simulink model "NAO68"  (R2021b)
settings: Solver=VariableStepAuto  StartTime=0.0  StopTime=2
undefined symbols (not defined in the file): foot_z, X, Y, Z
libraries: sm_lib x258, nesl_utility x25, Contact_Forces_Lib x3, simulink x1
(part 6 of 6)

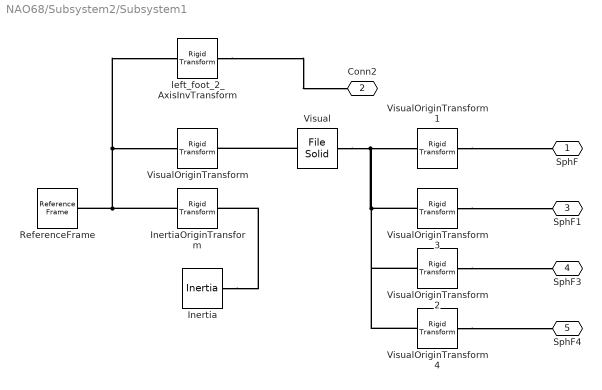
== system NAO68/Subsystem2/Subsystem1 ==
  Inertia : sm_lib/Body Elements/Inertia  InertiaType=Custom  Mass=2.1641e-17  MassUnits=kg  CenterOfMass=[0, 0, 0]  CenterOfMassUnits=m  MomentsOfInertia=[5.1574e-20, 4.4176e-20, 1.2071e-20]  MomentsOfInertiaUnits=kg*m^2  ProductsOfInertia=[-1.2733e-21, -1.1553e-22, 2.4046e-23]  ProductsOfInertiaUnits=kg*m^2  GraphicType=None  MarkerShape=Inertia  MarkerSize=20  GraphicVisPropType=SimpleVisualProperties  GraphicDiffuseColor=[0.5 0.5 0.5]  GraphicSpecularColor=[0.5 0.5 0.5 1.0]  GraphicAmbientColor=[0.15 0.15 0.15 1.0]  GraphicEmissiveColor=[0.0 0.0 0.0 1.0]  GraphicShininess=75  GraphicOpacity=1.0
  InertiaOriginTransform : sm_lib/Frames and Transforms/Rigid Transform  TranslationMethod=Cartesian  TranslationStandardOffset=0  TranslationLengthUnit=m  TranslationStandardAxis=+Z  TranslationCartesianOffset=[-0.0322560679316395, 0.00368111914052804, -0.031057785127505]  TranslationROffset=0  TranslationROffsetUnits=m  TranslationZOffset=0  TranslationZOffsetUnits=m  TranslationThetaOffset=0  TranslationThetaOffsetUnits=deg  RotationMethod=RotationSequence  RotationAngleUnits=deg  RotationStandardAxis=+Z  RotationAngle=0.0  RotationArbitraryAxis=[0 0 1]  FollAlignAxisA=+X  BaseAlignAxisA=+Y  FollAlignAxisB=+Y  BaseAlignAxisB=+Z  RotationSequenceAxes=BaseAxes  RotationSequence=XYZ  RotationSequenceAngles=[0, 0, 0]  RotationSequenceAnglesUnits=rad  RotationMatrix=[1 0 0; 0 1 0; 0 0 1]
  ReferenceFrame : sm_lib/Frames and Transforms/Reference Frame
  Visual : sm_lib/Body Elements/File Solid  ExtGeomFileName=NAO68/meshes/left foot.STL  UnitType=Custom  ExtGeomFileUnits=m  StepReaderType=HEX  ExportConvexHullGeometry=off  InertiaType=Custom  Mass=1  MassUnits=kg  CenterOfMass=[0, 0, 0]  CenterOfMassUnits=m  MomentsOfInertia=[0, 0, 0]  MomentsOfInertiaUnits=kg*m^2  ProductsOfInertia=[0, 0, 0]  ProductsOfInertiaUnits=kg*m^2  BasedOnType=DensityFromFile  Density=1000  DensityUnits=kg/m^3  DoExposeReferenceFrame=on  SerializedFrames=<Frames><Frame><Id>Frame1</Id><Value><Name>F1</Name><Origin><Source>ReferenceFrame</Source><FeatureName></FeatureName></Origin><PrimaryAxis><DefinedDirection>+Z</DefinedDirection><Source>ReferenceFrame</Source><SourceDirection>+X</SourceDirection><FeatureName></FeatureName></PrimaryAxis><SecondaryAxis><DefinedDirection>-X</DefinedDirection><Source>ReferenceFrame</Source><SourceDirection>-Z</SourceDirection><FeatureName></FeatureName></SecondaryAxis></Value></Frame></Frames>  GraphicType=FromGeometry  MarkerShape=Sphere  MarkerSize=10  GraphicVisPropType=SimpleVisualProperties  GraphicDiffuseColor=[0.79216, 0.8196099999999999, 0.93333]  GraphicSpecularColor=[0.5 0.5 0.5 1.0]  GraphicAmbientColor=[0.15 0.15 0.15 1.0]  GraphicEmissiveColor=[0.0 0.0 0.0 1.0]  GraphicShininess=75  GraphicOpacity=1
  VisualOriginTransform : sm_lib/Frames and Transforms/Rigid Transform  TranslationMethod=Cartesian  TranslationStandardOffset=0  TranslationLengthUnit=m  TranslationStandardAxis=+Z  TranslationCartesianOffset=[0, 0, 0]  TranslationROffset=0  TranslationROffsetUnits=m  TranslationZOffset=0  TranslationZOffsetUnits=m  TranslationThetaOffset=0  TranslationThetaOffsetUnits=deg  RotationMethod=RotationSequence  RotationAngleUnits=deg  RotationStandardAxis=+Z  RotationAngle=0.0  RotationArbitraryAxis=[0 0 1]  FollAlignAxisA=+X  BaseAlignAxisA=+Y  FollAlignAxisB=+Y  BaseAlignAxisB=+Z  RotationSequenceAxes=BaseAxes  RotationSequence=XYZ  RotationSequenceAngles=[0, 0, 0]  RotationSequenceAnglesUnits=rad  RotationMatrix=[1 0 0; 0 1 0; 0 0 1]
  VisualOriginTransform1 : sm_lib/Frames and Transforms/Rigid Transform  TranslationMethod=Cartesian  TranslationStandardOffset=0  TranslationLengthUnit=mm  TranslationStandardAxis=+Z  TranslationCartesianOffset=[-95,130, -36]  TranslationROffset=0  TranslationROffsetUnits=m  TranslationZOffset=0  TranslationZOffsetUnits=m  TranslationThetaOffset=0  TranslationThetaOffsetUnits=deg  RotationMethod=RotationSequence  RotationAngleUnits=deg  RotationStandardAxis=+Z  RotationAngle=0.0  RotationArbitraryAxis=[0 0 1]  FollAlignAxisA=+X  BaseAlignAxisA=+Y  FollAlignAxisB=+Y  BaseAlignAxisB=+Z  RotationSequenceAxes=BaseAxes  RotationSequence=XYZ  RotationSequenceAngles=[0, 0, 0]  RotationSequenceAnglesUnits=rad  RotationMatrix=[1 0 0; 0 1 0; 0 0 1]
  VisualOriginTransform2 : sm_lib/Frames and Transforms/Rigid Transform  TranslationMethod=Cartesian  TranslationStandardOffset=0  TranslationLengthUnit=mm  TranslationStandardAxis=+Z  TranslationCartesianOffset=[60,130, -36]  TranslationROffset=0  TranslationROffsetUnits=m  TranslationZOffset=0  TranslationZOffsetUnits=m  TranslationThetaOffset=0  TranslationThetaOffsetUnits=deg  RotationMethod=RotationSequence  RotationAngleUnits=deg  RotationStandardAxis=+Z  RotationAngle=0.0  RotationArbitraryAxis=[0 0 1]  FollAlignAxisA=+X  BaseAlignAxisA=+Y  FollAlignAxisB=+Y  BaseAlignAxisB=+Z  RotationSequenceAxes=BaseAxes  RotationSequence=XYZ  RotationSequenceAngles=[0, 0, 0]  RotationSequenceAnglesUnits=rad  RotationMatrix=[1 0 0; 0 1 0; 0 0 1]
  VisualOriginTransform3 : sm_lib/Frames and Transforms/Rigid Transform  TranslationMethod=Cartesian  TranslationStandardOffset=0  TranslationLengthUnit=mm  TranslationStandardAxis=+Z  TranslationCartesianOffset=[-95,-145, -36]  TranslationROffset=0  TranslationROffsetUnits=m  TranslationZOffset=0  TranslationZOffsetUnits=m  TranslationThetaOffset=0  TranslationThetaOffsetUnits=deg  RotationMethod=RotationSequence  RotationAngleUnits=deg  RotationStandardAxis=+Z  RotationAngle=0.0  RotationArbitraryAxis=[0 0 1]  FollAlignAxisA=+X  BaseAlignAxisA=+Y  FollAlignAxisB=+Y  BaseAlignAxisB=+Z  RotationSequenceAxes=BaseAxes  RotationSequence=XYZ  RotationSequenceAngles=[0, 0, 0]  RotationSequenceAnglesUnits=rad  RotationMatrix=[1 0 0; 0 1 0; 0 0 1]
  VisualOriginTransform4 : sm_lib/Frames and Transforms/Rigid Transform  TranslationMethod=Cartesian  TranslationStandardOffset=0  TranslationLengthUnit=mm  TranslationStandardAxis=+Z  TranslationCartesianOffset=[60,-145, -36]  TranslationROffset=0  TranslationROffsetUnits=m  TranslationZOffset=0  TranslationZOffsetUnits=m  TranslationThetaOffset=0  TranslationThetaOffsetUnits=deg  RotationMethod=RotationSequence  RotationAngleUnits=deg  RotationStandardAxis=+Z  RotationAngle=0.0  RotationArbitraryAxis=[0 0 1]  FollAlignAxisA=+X  BaseAlignAxisA=+Y  FollAlignAxisB=+Y  BaseAlignAxisB=+Z  RotationSequenceAxes=BaseAxes  RotationSequence=XYZ  RotationSequenceAngles=[0, 0, 0]  RotationSequenceAnglesUnits=rad  RotationMatrix=[1 0 0; 0 1 0; 0 0 1]
  left_foot_2_AxisInvTransform : sm_lib/Frames and Transforms/Rigid Transform  TranslationMethod=Cartesian  TranslationStandardOffset=0  TranslationLengthUnit=m  TranslationStandardAxis=+Z  TranslationCartesianOffset=[0, 0, 0]  TranslationROffset=0  TranslationROffsetUnits=m  TranslationZOffset=0  TranslationZOffsetUnits=m  TranslationThetaOffset=0  TranslationThetaOffsetUnits=deg  RotationMethod=ArbitraryAxis  RotationAngleUnits=rad  RotationStandardAxis=+Z  RotationAngle=3.141592653589793  RotationArbitraryAxis=[1, 0, 0]  FollAlignAxisA=+X  BaseAlignAxisA=+Y  FollAlignAxisB=+Y  BaseAlignAxisB=+Z  RotationSequenceAxes=FollowerAxes  RotationSequence=XYX  RotationSequenceAngles=[0 0 0]  RotationSequenceAnglesUnits=deg  RotationMatrix=[1 0 0; 0 1 0; 0 0 1]
  SphF : PMIOPort  Side=Right
  Conn2 : PMIOPort  Port=2  Side=Left
  SphF1 : PMIOPort  Port=3  Side=Right
  SphF3 : PMIOPort  Port=4  Side=Right
  SphF4 : PMIOPort  Port=5  Side=Right
  connections:
  InertiaOriginTransform/LConn1 -- ReferenceFrame/RConn1 -- VisualOriginTransform/LConn1 -- left_foot_2_AxisInvTransform/LConn1
  Inertia/RConn1 -- InertiaOriginTransform/RConn1
  left_foot_2_AxisInvTransform/RConn1 -- Conn2/RConn1
  Visual/RConn1 -- VisualOriginTransform/RConn1
  VisualOriginTransform1/RConn1 -- SphF/RConn1
  Visual/LConn1 -- VisualOriginTransform4/LConn1 -- VisualOriginTransform2/LConn1 -- VisualOriginTransform3/LConn1 -- VisualOriginTransform1/LConn1
  VisualOriginTransform3/RConn1 -- SphF1/RConn1
  VisualOriginTransform2/RConn1 -- SphF3/RConn1
  VisualOriginTransform4/RConn1 -- SphF4/RConn1

== matlab function NAO68/MATLAB Function1 ==
  data: x input; theta6 output; theta7 output; theta8 output; theta9 output; theta10 output; model input
function [theta6,theta7,theta8,theta9,theta10] = xyztoang(x,model)
 

 theta6=-2*asin(x/100);
 theta7=-pi/10;
 theta8=pi/2;
 theta9=-1.5*(theta6);
 if(theta9<0)
     theta9=0;
 elseif(model==3)
     theta8=pi/2;
     theta9=pi/2;
 end
theta10=-pi/2;

end

== matlab function NAO68/MATLAB Function ==
  data: x input; theta1 output; model input; theta2 output; theta3 output; theta4 output; theta5 output
function [theta1,theta2,theta3,theta4,theta5] = xyztoang(x,model)

 theta1=2*asin(x/100);
 theta2=-pi/10;
 theta3=-pi/2;
 theta4=1.5*(theta1);
 if(theta4<0)
     theta4=0;
 elseif(model==3)
     theta4=pi/2;
 end
 theta5=-pi/2;


end

== matlab function NAO68/MATLAB Function2 ==
  data: theta11 output; theta12 output
function [ theta11,theta12] = xyztoang

theta11=0;
theta12=0;

end

== matlab function NAO68/MATLAB Function3 ==
  data: theta19 output; theta20 output; theta21 output; theta22 output; theta23 output; theta24 output; t1 input; model input
function [theta19,theta20,theta21,theta22,theta23,theta24] = fcn(t1,model)
 
l1=100;
l2=102.75+45;
 
if(model==1)&&(0<=t1)&&(t1<=1) 
%     theta24=-0.9*t1/pi;
    theta24=0;

    theta19=0;
    theta20=0;
    theta21=0;
    theta22=0;
    theta23=0;
elseif(model==1)&&(1<t1)&&(t1<=2)
     theta23=(1-t1)/pi;
%      theta24=-0.9*(2-t1)/pi;
      theta24=0;
     theta19=0;
     theta20=0;
     theta21=0;
     theta22=0;
elseif(model==1)&&(t1>2)&&(t1<=2.5)
    theta24=0;
    theta19=0;
    theta20=0;
    theta21=3*(2-t1)*asin(50/l1);
    theta22=3*(t1-2)*asin(50/l1);
    theta23=2*(t1-2.5)/pi;
elseif(model==1)&&(t1>2.5)&&(t1<=3)
    theta24=0;
    theta19=0;
    theta20=0;
    theta21=-1.5*asin(50/l1);
    theta22=1.5/((t1-1.5)/1)*asin(50/l1);
    theta23=0;
elseif(model==1)&&(t1>3)&&(t1<=3.5)
    theta24=0;
    theta19=0;
    theta20=0;
    theta21=-1.5*asin(50/l1);
    theta22=asin(50/l1);
    theta23=0;
elseif(model==1)&&(t1>3.5)&&(t1<=4)
    theta24=0;
    theta19=0;
    theta20=0;
    theta21=-1.5*asin(50/l1);
    theta22=asin(50/l1);
    theta23=0;
elseif(model==1)&&(t1>4)&&(t1<=4.5)
    theta24=0;
    theta19=0;
    theta20=0;
    theta21=-3*(4.5-t1)*asin(50/l1);
    theta22=2*(4.5-t1)*asin(50/l1);
    theta23=0;
 
%kicking
elseif(model==2)&&(0<=t1)&&(t1<0.5)
    theta19=0;
    theta20=0;
    theta21=-2.5*t1*asin(50/l1);
    theta22=2.5*t1*asin(50/l1);
    theta23=0;
    theta24=0;
    elseif(model==2)&&(0.5<=t1)&&(t1<=1)
    theta19=0;
    theta20=0;
    theta21=-1.25*asin(50/l1);
    theta22=2.5*(1-t1)*asin(50/l1);
    theta23=0;
    theta24=0;
    elseif(model==2)&&(1<t1)&&(t1<=1.5)
    theta19=0;
    theta20=0;
    theta21=-1.25*asin(50/l1);
    theta22=-2.5*(1-t1)*asin(50/l1);
    theta23=0;
    theta24=0;
    elseif(model==2)&&(1.5<t1)&&(t1<=2)
    theta19=0;
    theta20=0;
    theta21=-2.5*(2-t1)*asin(50/l1);
    theta22=2.5*(2-t1)*asin(50/l1);
    theta23=0;
    theta24=0;

 %turn right
    elseif(model==3)&&(t1>=0)&&(t1<0.5)
    theta19=0;
    theta20=0;
    theta21=-2*t1*asin(0.5);
    theta22=4.5*t1*asin(0.5);
    theta23=-theta22-theta21;
    theta24=0;
    elseif(model==3)&&(t1>=0.5)&&(t1<=1)
    theta19=0;
    theta20=-1.5*(t1-0.5)*asin(0.5);
    theta21=-2*0.5*asin(0.5);
    theta22=4.5*0.5*asin(0.5);
    theta23=-theta22-theta21;
    theta24=1.5*(t1-0.5)*asin(0.5);
    elseif(model==3)&&(t1>1)&&(t1<=1.5)
    theta19=-pi*(t1-1);
    theta20=-1.5*asin(0.5)*0.5;
    theta21=-2*0.5*asin(0.5)-(t1-1)*asin(0.5);
    theta22=4.5*0.5*asin(0.5)+2*(t1-1)*asin(0.5);
    theta23=-2.5*asin(0.5)*(1.5-t1);
    theta24=1.5*asin(0.5)*(1.5-t1);
    elseif(model==3)&&(t1>1.5)&&(t1<=2)
    theta19=-pi*0.5;
    theta20=-1.5*asin(0.5)*0.5;
    theta21=-1.5*asin(0.5);
    theta22=3.25*asin(0.5);
    theta23=0;
    theta24=0;
    else 
    theta19=0;
    theta20=0;
    theta21=0;
    theta22=0;
    theta23=0;
    theta24=0;
end



end

== matlab function NAO68/MATLAB Function4 ==
  data: theta13 output; theta14 output; theta15 output; theta16 output; theta17 output; theta18 output; t2 input; model input
 
function [theta13,theta14,theta15,theta16,theta17,theta18]=fcn(t2,model)
    l1=100;
    l2=102.75;

%walking 
if(model==1)&&(0<=t2)&&(t2<0.5)
    theta13=0;
    theta14=0;
    theta15=3*t2*asin(50/l1);
    theta16=3*t2*asin(50/l1);
    theta17=0;
    theta18=0;

elseif(model==1)&&(0.5<=t2)&&(t2<=1)
    theta13=0;
    theta14=0;
    theta15=1.5*asin(50/l1);
    theta16=1.5*asin(50/l1);
    theta17=0;
    theta18=0;
elseif(model==1)&&(t2>1)&&(t2<=1.5)
    theta13=0;
    theta14=0;
    theta15=1.5*asin(50/l1);
    theta16=(1/t2)*1.5*asin(50/l1);
    theta17=0;
    theta18=0;
    elseif(model==1)&&(t2>1.5)&&(t2<=2)
    theta13=0;
    theta14=0;
    theta15=1.5*asin(50/l1);
    theta16=asin(50/l1);
    theta17=0;
    theta18=0;
    elseif(model==1)&&(2<t2)&&(t2<=2.5)
    theta13=0;
    theta14=0;
    theta15=3*(2.5-t2)*asin(50/l1);
    theta16=2*(2.5-t2)*asin(50/l1);
    theta17=0;
    theta18=0;
%     theta18=0.9*(t2-2)/pi;
    elseif(model==1)&&(2.5<t2)&&(t2<=3)
    theta13=0;
    theta14=0;
    theta15=0;
    theta16=0;
    theta17=0;
    theta18=0;
%     theta18=0.9*(t2-2)/pi;
    elseif(model==1)&&(t2>3)&&(t2<=3.5)
    theta13=0;
    theta14=0;
    theta15=0;
    theta16=0;
    theta17=(t2-3)/pi;
    theta18=0;
%     theta18=1.8*(3.5-t2)/pi;
    elseif(model==1)&&(t2>3.5)&&(t2<=4)
    theta13=0;
    theta14=0;
    theta15=0;
    theta16=0;
    theta17=(t2-3)/pi;
    theta18=0;
    elseif(model==1)&&(t2>4)&&(t2<=4.5)
    theta13=0;
    theta14=0;
    theta15=0;
    theta16=0;
    theta17=2*(4.5-t2)/pi;
    theta18=0;

%     theta13=0;
%     theta14=0;
%     theta15=0;
%     theta16=0;
%     theta17=0;
%     theta18=0;

%kicking
elseif(model==2)
    theta13=0;
    theta14=0;
    theta15=0;
    theta16=0;
    theta17=0;
    theta18=0;

%turn right
    elseif(model==3)&&(t2>=0)&&(t2<0.5)
    theta13=0;
    theta14=0;
    theta15=2*t2*asin(0.5);
    theta16=4.5*t2*asin(0.5);
    theta17=theta16-theta15;
    theta18=0;
    elseif(model==3)&&(t2>=0.5)&&(t2<1)
    theta13=0;
    theta14=-1.5*(t2-0.5)*asin(0.5);
    theta15=1*asin(0.5);
    theta16=2.25*asin(0.5);
    theta17=theta16-theta15;
    theta18=1.5*(t2-0.5)*asin(0.5);
     elseif(model==3)&&(t2>=1)&&(t2<1.5)
    theta13=0;
    theta14=-0.75*asin(0.5);
    theta15=1*asin(0.5);
    theta16=2.25*asin(0.5);
    theta17=theta16-theta15;
    theta18=0.75*asin(0.5);
     elseif(model==3)&&(t2>=1.5)&&(t2<2)
    theta13=0;
    theta14=-0.75*asin(0.5);
    theta15=1*asin(0.5);
    theta16=2.25*asin(0.5);
    theta17=theta16-theta15;
    theta18=0.75*asin(0.5);
else
    theta13=0;
    theta14=0;
    theta15=0;
    theta16=0;
    theta17=0;
    theta18=0;


end

== matlab function NAO68/MATLAB Function5 ==
  data: model input; y output; x input
function y = fcn(model,x)
if(model==1)
    y=x;
elseif(model==2)
    y=0;
elseif(model==3)
    y=0;
else
    y=x;
   

end
